simulink model "GolfSwingZVCF"  (R2024b)
settings: Solver=VariableStepAuto  StartTime=0.0  StopTime=StopTime  MaxStep=0.001  RelTol=1e-3
PreLoadFcn:
  | cd(matlabdrive);
  | cd '2DModel';
PostLoadFcn:
  | %run SCRIPT_mdlWksGenerate.m;
  | mdlWks=get_param('GolfSwingZVCF','ModelWorkspace');
  | mdlWks.DataSource = 'MAT-File';
  | mdlWks.FileName = 'ModelInputs.mat';
  | mdlWks.reload;
model workspace: external: MAT-File ModelInputsZVCF.mat (data not in the file)
undefined symbols (not defined in the file): JointTorqueHip, JointTorqueLElbow, JointTorqueLScap, JointTorqueLShoulder, JointTorqueLWrist, JointTorqueRElbow, JointTorqueRScap, JointTorqueRShoulder, JointTorqueRWrist, JointTorqueTorso, X, Y, Z
libraries: nesl_utility x286, sm_lib x176, matrix_library x11, simulink_extras x2
(part 3 of 9)

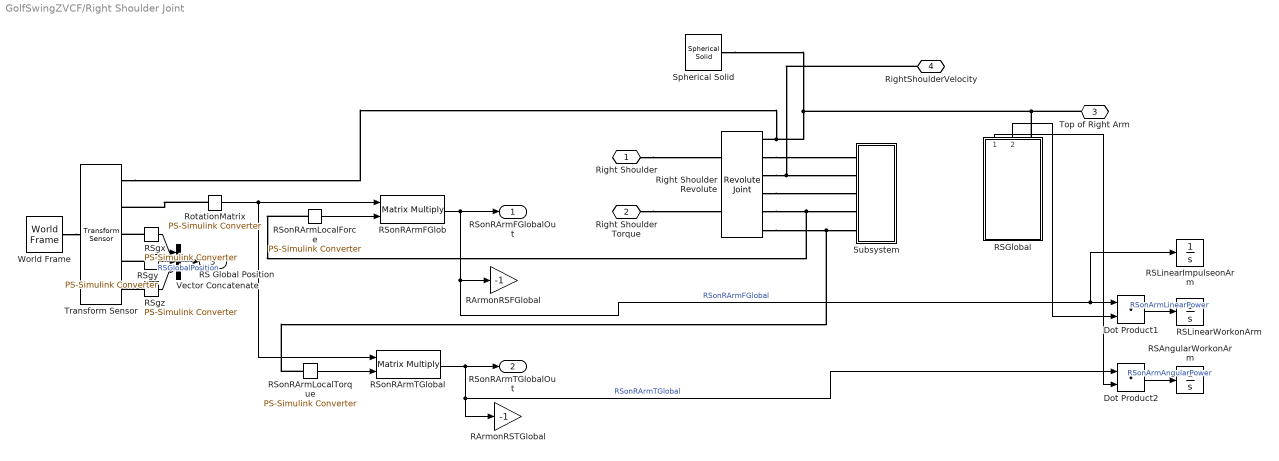
== system GolfSwingZVCF/Right Shoulder Joint ==
  Dot Product1 : DotProduct  OutDataTypeStr=Inherit: Inherit via internal rule
  Dot Product2 : DotProduct  OutDataTypeStr=Inherit: Inherit via internal rule
  RArmonRSFGlobal : Gain  Gain=-1
  RArmonRSTGlobal : Gain  Gain=-1
  RSAngularWorkonArm : Integrator
  RSGlobal : Subsystem
  RSLinearImpulseonArm : Integrator
  RSLinearWorkonArm : Integrator
  RSgx : nesl_utility/PS-Simulink Converter  PhysicalDomain=network_engine_domain  SubClassName=ps_output  LeftPortType=input  RightPortType=output  PseudoPeriodic=off  Frequencies=[]  VectorFormat=1-D array  Unit=inherit  AffineConversion=off
  RSgy : nesl_utility/PS-Simulink Converter  PhysicalDomain=network_engine_domain  SubClassName=ps_output  LeftPortType=input  RightPortType=output  PseudoPeriodic=off  Frequencies=[]  VectorFormat=1-D array  Unit=inherit  AffineConversion=off
  RSgz : nesl_utility/PS-Simulink Converter  PhysicalDomain=network_engine_domain  SubClassName=ps_output  LeftPortType=input  RightPortType=output  PseudoPeriodic=off  Frequencies=[]  VectorFormat=1-D array  Unit=inherit  AffineConversion=off
  RSonRArmFGlob : Product  Multiplication=Matrix(*)
  RSonRArmLocalForce : nesl_utility/PS-Simulink Converter  PhysicalDomain=network_engine_domain  SubClassName=ps_output  LeftPortType=input  RightPortType=output  PseudoPeriodic=off  Frequencies=[]  VectorFormat=1-D array  Unit=inherit  AffineConversion=off
  RSonRArmLocalTorque : nesl_utility/PS-Simulink Converter  PhysicalDomain=network_engine_domain  SubClassName=ps_output  LeftPortType=input  RightPortType=output  PseudoPeriodic=off  Frequencies=[]  VectorFormat=1-D array  Unit=inherit  AffineConversion=off
  RSonRArmTGlobal : Product  Multiplication=Matrix(*)
  Right Shoulder Revolute : sm_lib/Joints/Revolute Joint  JointMode=Normal  CompositeWrenchDir=BaseOnFollower  CompositeWrenchFrame=FollowerFrame  SenseConstraintForce=off  SenseConstraintTorque=off  SenseTotalForce=on  SenseTotalTorque=on  PositionTargetSpecify=on  PositionTargetPriority=Low  PositionTargetValue=RShoulderStartPosition  PositionTargetValueUnits=deg  VelocityTargetSpecify=on  VelocityTargetPriority=High  VelocityTargetValue=RShoulderStartVelocity  VelocityTargetValueUnits=deg/s  EquilibriumPosition=0  EquilibriumPositionUnits=deg  SpringStiffness=0  SpringStiffnessUnits=N*m/deg  DampingCoefficient=0  DampingCoefficientUnits=N*m/(deg/s)  LowerLimitSpecify=off  LowerLimitBound=-150  LowerLimitBoundUnits=deg  LowerLimitStiffness=1e4  LowerLimitStiffnessUnits=N*m/deg  LowerLimitDamping=10  LowerLimitDampingUnits=N*m/(deg/s)  LowerLimitTransitionRegionWidth=0.1  LowerLimitTransitionRegionWidthUnits=deg  UpperLimitSpecify=off  UpperLimitBound=65  UpperLimitBoundUnits=deg  UpperLimitStiffness=1e4  UpperLimitStiffnessUnits=N*m/deg  UpperLimitDamping=10  UpperLimitDampingUnits=N*m/(deg/s)  UpperLimitTransitionRegionWidth=0.1  UpperLimitTransitionRegionWidthUnits=deg  TorqueActuationMode=InputTorque  MotionActuationMode=ComputedMotion  SensePosition=on  SenseVelocity=on  SenseAcceleration=on  SenseTorqueForce=off  SenseLowerLimitTorqueForce=off  SenseUpperLimitTorqueForce=off
      settings: LogSimulationData=on
  RotationMatrix : nesl_utility/PS-Simulink Converter  PhysicalDomain=network_engine_domain  SubClassName=ps_output  LeftPortType=input  RightPortType=output  PseudoPeriodic=off  Frequencies=[]  VectorFormat=1-D array  Unit=inherit  AffineConversion=off
  Spherical Solid : sm_lib/Body Elements/Spherical Solid  SphereRadius=1.75  SphereRadiusUnits=in  ExportEntireGeometry=off  InertiaType=CalculateFromGeometry  BasedOnType=Density  Density=0  DensityUnits=kg/m^3  Mass=1  MassUnits=kg  CenterOfMass=[0 0 0]  CenterOfMassUnits=m  MomentsOfInertia=[1 1 1]  MomentsOfInertiaUnits=kg*m^2  ProductsOfInertia=[0 0 0]  ProductsOfInertiaUnits=kg*m^2  GraphicType=FromGeometry  MarkerShape=Sphere  MarkerSize=10  GraphicVisPropType=SimpleVisualProperties  GraphicDiffuseColor=[0.2 0.2 1.0]  GraphicOpacity=1  GraphicSpecularColor=[0.5 0.5 0.5 1.0]  GraphicAmbientColor=[0.15 0.15 0.15 1.0]  GraphicEmissiveColor=[0.0 0.0 0.0 1.0]  GraphicShininess=75  DoExposeReferenceFrame=on  SerializedFrames=<Frames/>
  Subsystem : Subsystem
  Transform Sensor : sm_lib/Frames and Transforms/Transform Sensor  MeasurementFrame=World  RotationSequence=XYX  SenseAngle=off  SenseAxis=off  SenseQ=off  SenseR=on  SenseRotationSequence=off  SenseOmegaX=off  SenseOmegaY=off  SenseOmegaZ=off  SenseOmega=off  SenseQDot=off  SenseRDot=off  SenseRotationSequenceDot=off  SenseAlphaX=off  SenseAlphaY=off  SenseAlphaZ=off  SenseAlpha=off  SenseQDDot=off  SenseRDDot=off  SenseX=on  SenseY=on  SenseZ=on  SenseXYZ=off  SenseRad=off  SenseAzim=off  SenseDist=off  SenseInc=off  SenseXDot=off  SenseYDot=off  SenseZDot=off  SenseXYZDot=off  SenseRadDot=off  SenseAzimDot=off  SenseDistDot=off  SenseIncDot=off  SenseXDDot=off  SenseYDDot=off  SenseZDDot=off  SenseXYZDDot=off  SenseRadDDot=off  SenseAzimDDot=off  SenseDistDDot=off  SenseIncDDot=off
  Vector Concatenate : Concatenate  NumInputs=3
  World Frame : sm_lib/Frames and Transforms/World Frame
  Right Shoulder : PMIOPort  Side=Left
  Right Shoulder Torque : PMIOPort  Port=2  Side=Left
  Top of Right Arm : PMIOPort  Port=3  Side=Right
  RightShoulderVelocity : PMIOPort  Port=4  Side=Right
  RSonRArmFGlobalOut : Outport
  RSonRArmTGlobalOut : Outport  Port=2
  RS Global Position : Outport  Port=3
  wires:
  RotationMatrix/1 -> RSonRArmFGlob/1, RSonRArmTGlobal/1
  RSonRArmLocalForce/1 -> RSonRArmFGlob/2
  RSonRArmLocalTorque/1 -> RSonRArmTGlobal/2
  RSonRArmTGlobal/1 -> Dot Product2/1, RArmonRSTGlobal/1, RSonRArmTGlobalOut/1  "RSonRArmTGlobal"
  RSgx/1 -> Vector Concatenate/1
  RSgy/1 -> Vector Concatenate/2
  Vector Concatenate/1 -> RS Global Position/1  "RSGlobalPosition"
  RSgz/1 -> Vector Concatenate/3
  Dot Product1/1 -> RSLinearWorkonArm/1  "RSonArmLinearPower"
  Dot Product2/1 -> RSAngularWorkonArm/1  "RSonArmAngularPower"
  RSGlobal/1(RightShoulderGlobalAV) -> Dot Product2/2
  RSGlobal/2(RightShoulderGlobalVelocity) -> Dot Product1/2
  RSonRArmFGlob/1 -> RSLinearImpulseonArm/1, Dot Product1/1, RArmonRSFGlobal/1, RSonRArmFGlobalOut/1  "RSonRArmFGlobal"
  connections:
  Right Shoulder Revolute/RConn6 -- RSonRArmLocalTorque/LConn1 -- Subsystem/LConn5
  Right Shoulder Revolute/RConn4 -- Subsystem/LConn3
  Right Shoulder Revolute/RConn2 -- Subsystem/LConn1
  Right Shoulder Revolute/RConn5 -- RSonRArmLocalForce/LConn1 -- Subsystem/LConn4
  Right Shoulder Revolute/RConn3 -- RightShoulderVelocity/RConn1 -- Subsystem/LConn2
  Right Shoulder Torque/RConn1 -- Right Shoulder Revolute/LConn2
  Right Shoulder/RConn1 -- Right Shoulder Revolute/LConn1
  Spherical Solid/RConn1 -- Top of Right Arm/RConn1 -- RSGlobal/RConn1 -- Transform Sensor/RConn1 -- Right Shoulder Revolute/RConn1
  RSgx/LConn1 -- Transform Sensor/RConn3
  RotationMatrix/LConn1 -- Transform Sensor/RConn2
  RSgz/LConn1 -- Transform Sensor/RConn5
  RSgy/LConn1 -- Transform Sensor/RConn4
  World Frame/RConn1 -- Transform Sensor/LConn1

== system GolfSwingZVCF/Right Upper Arm MOF ==
  RS Global Position : Inport
  RE Global Position : Inport  Port=2
  RSonRArmFGlobalIn : Inport  Port=3
  RSonRArmTGlobalIn : Inport  Port=4
  RForearmonRArmFGlobalIn : Inport  Port=5
  RForearmonRArmTGlobalIn : Inport  Port=6
  R Vector Elbow Force on Right Arm : Sum  Inputs=-+
  R Vector Shoulder Force on Right Arm : Sum  Inputs=-+
  RElbowonRArmMOFGlobal : matrix_library/Cross Product
  RElbowonRArmMOFLocal : Product  Multiplication=Matrix(*)
  RSAngularImpulseonArm : Integrator
  RShoulderonRArmMOFGlobal : matrix_library/Cross Product
  RShoulderonRArmMOFLocal : Product  Multiplication=Matrix(*)
  RUACOM : sm_lib/Body Elements/Inertia Sensor  SensorExtent=BodyGroup  SpanWeldJoints=off  ExcludeGroundedBodies=off  MeasurementFrame=World  SenseMass=off  SenseCenterOfMass=on  SenseInertiaMatrix=off  SenseCenteredInertiaMatrix=off  SensePrincipalInertiaMatrix=off  SenseRotationMatrix=off  GraphicType=None  PrincipalInertiaFrameSize=20  GraphicVisPropType=SimpleVisualProperties  GraphicDiffuseColor=[0.5 0.5 0.5]  GraphicOpacity=1  GraphicSpecularColor=[0.5 0.5 0.5 1.0]  GraphicAmbientColor=[0.15 0.15 0.15 1.0]  GraphicEmissiveColor=[0.0 0.0 0.0 1.0]  GraphicShininess=75
  Right Upper Arm COM : nesl_utility/PS-Simulink Converter  PhysicalDomain=network_engine_domain  SubClassName=ps_output  LeftPortType=input  RightPortType=output  PseudoPeriodic=off  Frequencies=[]  VectorFormat=1-D array  Unit=inherit  AffineConversion=off
  Rotation Transform Right Arm : nesl_utility/PS-Simulink Converter  PhysicalDomain=network_engine_domain  SubClassName=ps_output  LeftPortType=input  RightPortType=output  PseudoPeriodic=off  Frequencies=[]  VectorFormat=1-D array  Unit=inherit  AffineConversion=off
  SumofMomentsRArmLocal : Product  Multiplication=Matrix(*)
  SumofMomentsRSonRArm : Sum
  SumofMomentsRightArmGlobal : Sum  Inputs=++++
  Transform Sensor : sm_lib/Frames and Transforms/Transform Sensor  MeasurementFrame=World  RotationSequence=XYX  SenseAngle=off  SenseAxis=off  SenseQ=off  SenseR=on  SenseRotationSequence=off  SenseOmegaX=off  SenseOmegaY=off  SenseOmegaZ=off  SenseOmega=off  SenseQDot=off  SenseRDot=off  SenseRotationSequenceDot=off  SenseAlphaX=off  SenseAlphaY=off  SenseAlphaZ=off  SenseAlpha=off  SenseQDDot=off  SenseRDDot=off  SenseX=off  SenseY=off  SenseZ=off  SenseXYZ=off  SenseRad=off  SenseAzim=off  SenseDist=off  SenseInc=off  SenseXDot=off  SenseYDot=off  SenseZDot=off  SenseXYZDot=off  SenseRadDot=off  SenseAzimDot=off  SenseDistDot=off  SenseIncDot=off  SenseXDDot=off  SenseYDDot=off  SenseZDDot=off  SenseXYZDDot=off  SenseRadDDot=off  SenseAzimDDot=off  SenseDistDDot=off  SenseIncDDot=off
  World Frame : sm_lib/Frames and Transforms/World Frame
  RightUpper  Arm : PMIOPort  Side=Left
  wires:
  Right Upper Arm COM/1 -> R Vector Elbow Force on Right Arm/1, R Vector Shoulder Force on Right Arm/1  "RUpperArmCOM"
  RS Global Position/1 -> R Vector Shoulder Force on Right Arm/2
  RE Global Position/1 -> R Vector Elbow Force on Right Arm/2
  RSonRArmFGlobalIn/1 -> RShoulderonRArmMOFGlobal/2
  R Vector Elbow Force on Right Arm/1 -> RElbowonRArmMOFGlobal/1
  RForearmonRArmTGlobalIn/1 -> SumofMomentsRightArmGlobal/4
  RForearmonRArmFGlobalIn/1 -> RElbowonRArmMOFGlobal/2
  R Vector Shoulder Force on Right Arm/1 -> RShoulderonRArmMOFGlobal/1
  SumofMomentsRightArmGlobal/1 -> SumofMomentsRArmLocal/2  "SumofMomentsRightArmGlobal"
  RElbowonRArmMOFGlobal/1 -> RElbowonRArmMOFLocal/2, SumofMomentsRightArmGlobal/2  "RElbowonRArmMOFGlobal"
  Rotation Transform Right Arm/1 -> SumofMomentsRArmLocal/1, RElbowonRArmMOFLocal/1, RShoulderonRArmMOFLocal/1
  RShoulderonRArmMOFGlobal/1 -> SumofMomentsRightArmGlobal/1, SumofMomentsRSonRArm/2, RShoulderonRArmMOFLocal/2  "RShoulderonRArmMOFGlobal"
  SumofMomentsRSonRArm/1 -> RSAngularImpulseonArm/1  "SumofMomentsRSonRArm"
  RSonRArmTGlobalIn/1 -> SumofMomentsRSonRArm/1, SumofMomentsRightArmGlobal/3
  connections:
  RUACOM/LConn1 -- Transform Sensor/LConn1 -- RightUpper  Arm/RConn1
  Right Upper Arm COM/LConn1 -- RUACOM/RConn1
  Transform Sensor/RConn1 -- World Frame/RConn1
  Rotation Transform Right Arm/LConn1 -- Transform Sensor/RConn2

== system GolfSwingZVCF/Right Wrist Joint ==
  ClubonRWFGlobal : Gain  Gain=-1
  ClubonRWTGlobal : Gain  Gain=-1
  RWLocalForce : nesl_utility/PS-Simulink Converter  PhysicalDomain=network_engine_domain  SubClassName=ps_output  LeftPortType=input  RightPortType=output  PseudoPeriodic=off  Frequencies=[]  VectorFormat=1-D array  Unit=inherit  AffineConversion=off
  RWLocalTorque : nesl_utility/PS-Simulink Converter  PhysicalDomain=network_engine_domain  SubClassName=ps_output  LeftPortType=input  RightPortType=output  PseudoPeriodic=off  Frequencies=[]  VectorFormat=1-D array  Unit=inherit  AffineConversion=off
  RWgx : nesl_utility/PS-Simulink Converter  PhysicalDomain=network_engine_domain  SubClassName=ps_output  LeftPortType=input  RightPortType=output  PseudoPeriodic=off  Frequencies=[]  VectorFormat=1-D array  Unit=inherit  AffineConversion=off
  RWgy : nesl_utility/PS-Simulink Converter  PhysicalDomain=network_engine_domain  SubClassName=ps_output  LeftPortType=input  RightPortType=output  PseudoPeriodic=off  Frequencies=[]  VectorFormat=1-D array  Unit=inherit  AffineConversion=off
  RWgz : nesl_utility/PS-Simulink Converter  PhysicalDomain=network_engine_domain  SubClassName=ps_output  LeftPortType=input  RightPortType=output  PseudoPeriodic=off  Frequencies=[]  VectorFormat=1-D array  Unit=inherit  AffineConversion=off
  RWonClubFGlobal : Product  Multiplication=Matrix(*)
  RWonClubTGlobal : Product  Multiplication=Matrix(*)
  Right Wrist : sm_lib/Joints/Revolute Joint  JointMode=Normal  CompositeWrenchDir=BaseOnFollower  CompositeWrenchFrame=FollowerFrame  SenseConstraintForce=off  SenseConstraintTorque=off  SenseTotalForce=on  SenseTotalTorque=on  PositionTargetSpecify=off  PositionTargetPriority=Low  PositionTargetValue=70  PositionTargetValueUnits=deg  VelocityTargetSpecify=off  VelocityTargetPriority=Low  VelocityTargetValue=0  VelocityTargetValueUnits=deg/s  EquilibriumPosition=0  EquilibriumPositionUnits=deg  SpringStiffness=0  SpringStiffnessUnits=N*m/deg  DampingCoefficient=0  DampingCoefficientUnits=N*m/(deg/s)  LowerLimitSpecify=off  LowerLimitBound=-90  LowerLimitBoundUnits=deg  LowerLimitStiffness=1e4  LowerLimitStiffnessUnits=N*m/deg  LowerLimitDamping=10  LowerLimitDampingUnits=N*m/(deg/s)  LowerLimitTransitionRegionWidth=0.1  LowerLimitTransitionRegionWidthUnits=deg  UpperLimitSpecify=off  UpperLimitBound=90  UpperLimitBoundUnits=deg  UpperLimitStiffness=1e4  UpperLimitStiffnessUnits=N*m/deg  UpperLimitDamping=10  UpperLimitDampingUnits=N*m/(deg/s)  UpperLimitTransitionRegionWidth=0.1  UpperLimitTransitionRegionWidthUnits=deg  TorqueActuationMode=InputTorque  MotionActuationMode=ComputedMotion  SensePosition=on  SenseVelocity=on  SenseAcceleration=on  SenseTorqueForce=off  SenseLowerLimitTorqueForce=off  SenseUpperLimitTorqueForce=off
      settings: LogSimulationData=on
  RightWristOutputs : Subsystem
  RightWristRelease : Subsystem  Commented=on
  RotationMatrix : nesl_utility/PS-Simulink Converter  PhysicalDomain=network_engine_domain  SubClassName=ps_output  LeftPortType=input  RightPortType=output  PseudoPeriodic=off  Frequencies=[]  VectorFormat=1-D array  Unit=inherit  AffineConversion=off
  Spherical Solid : sm_lib/Body Elements/Spherical Solid  SphereRadius=2  SphereRadiusUnits=in  ExportEntireGeometry=off  InertiaType=CalculateFromGeometry  BasedOnType=Density  Density=0  DensityUnits=kg/m^3  Mass=1  MassUnits=kg  CenterOfMass=[0 0 0]  CenterOfMassUnits=m  MomentsOfInertia=[1 1 1]  MomentsOfInertiaUnits=kg*m^2  ProductsOfInertia=[0 0 0]  ProductsOfInertiaUnits=kg*m^2  GraphicType=FromGeometry  MarkerShape=Sphere  MarkerSize=10  GraphicVisPropType=SimpleVisualProperties  GraphicDiffuseColor=[1.0 0.8 0.4]  GraphicOpacity=1  GraphicSpecularColor=[0.5 0.5 0.5 1.0]  GraphicAmbientColor=[0.15 0.15 0.15 1.0]  GraphicEmissiveColor=[0.0 0.0 0.0 1.0]  GraphicShininess=75  DoExposeReferenceFrame=on  SerializedFrames=<Frames/>
  Transform Sensor1 : sm_lib/Frames and Transforms/Transform Sensor  MeasurementFrame=World  RotationSequence=XYX  SenseAngle=off  SenseAxis=off  SenseQ=off  SenseR=on  SenseRotationSequence=off  SenseOmegaX=off  SenseOmegaY=off  SenseOmegaZ=off  SenseOmega=off  SenseQDot=off  SenseRDot=off  SenseRotationSequenceDot=off  SenseAlphaX=off  SenseAlphaY=off  SenseAlphaZ=off  SenseAlpha=off  SenseQDDot=off  SenseRDDot=off  SenseX=on  SenseY=on  SenseZ=on  SenseXYZ=off  SenseRad=off  SenseAzim=off  SenseDist=off  SenseInc=off  SenseXDot=off  SenseYDot=off  SenseZDot=off  SenseXYZDot=off  SenseRadDot=off  SenseAzimDot=off  SenseDistDot=off  SenseIncDot=off  SenseXDDot=off  SenseYDDot=off  SenseZDDot=off  SenseXYZDDot=off  SenseRadDDot=off  SenseAzimDDot=off  SenseDistDDot=off  SenseIncDDot=off
  Vector Concatenate : Concatenate  NumInputs=3
  World Frame1 : sm_lib/Frames and Transforms/World Frame
  Bottom of Right Forearm : PMIOPort  Side=Left
  RWForce : PMIOPort  Port=2  Side=Right
  RHGrip : PMIOPort  Port=3  Side=Right
  RWTorque : PMIOPort  Port=4  Side=Right
  Right Wrist Torque : PMIOPort  Port=5  Side=Right
  RWVelocity : PMIOPort  Port=6  Side=Right
  RWonClubTGlobalOut : Outport
  RWonClubFGlobalOut : Outport  Port=2
  ClubonRWFGlobalOut : Outport  Port=3
  ClubonRWTGlobalOut : Outport  Port=4
  RWGlobal Position : Outport  Port=5
  wires:
  RWLocalForce/1 -> RWonClubFGlobal/2
  RotationMatrix/1 -> RWonClubTGlobal/1, RWonClubFGlobal/1
  RWLocalTorque/1 -> RWonClubTGlobal/2
  ClubonRWFGlobal/1 -> ClubonRWFGlobalOut/1  "ClubonRWFGlobal"
  RWonClubFGlobal/1 -> ClubonRWFGlobal/1, RWonClubFGlobalOut/1  "RWonClubFGlobal"
  RWonClubTGlobal/1 -> ClubonRWTGlobal/1, RWonClubTGlobalOut/1  "RWonClubTGlobal"
  ClubonRWTGlobal/1 -> ClubonRWTGlobalOut/1  "ClubonRWTGlobal"
  RWgx/1 -> Vector Concatenate/1
  RWgz/1 -> Vector Concatenate/3
  Vector Concatenate/1 -> RWGlobal Position/1  "RWGlobalPosition"
  RWgy/1 -> Vector Concatenate/2
  connections:
  Right Wrist/RConn3 -- RWVelocity/RConn1 -- RightWristOutputs/LConn2
  Bottom of Right Forearm/RConn1 -- Spherical Solid/RConn1 -- Right Wrist/LConn1
  Right Wrist/RConn4 -- RightWristOutputs/LConn3
  Right Wrist/RConn1 -- Transform Sensor1/RConn1 -- RHGrip/RConn1
  Right Wrist/RConn2 -- RightWristOutputs/LConn1
  Right Wrist Torque/RConn1 -- Right Wrist/LConn2
  Right Wrist/RConn5 -- RWLocalForce/LConn1 -- RWForce/RConn1 -- RightWristOutputs/LConn4
  Right Wrist/RConn6 -- RightWristOutputs/LConn5 -- RWLocalTorque/LConn1 -- RWTorque/RConn1
  RotationMatrix/LConn1 -- Transform Sensor1/RConn2
  World Frame1/RConn1 -- Transform Sensor1/LConn1
  Transform Sensor1/RConn4 -- RWgy/LConn1
  Transform Sensor1/RConn5 -- RWgz/LConn1
  Transform Sensor1/RConn3 -- RWgx/LConn1

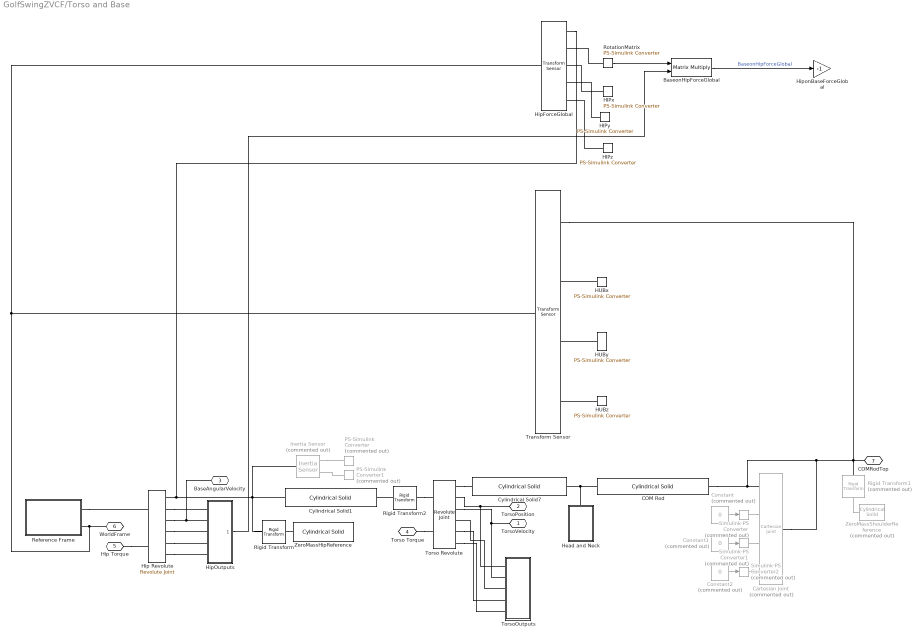
== system GolfSwingZVCF/Torso and Base ==
  BaseonHipForceGlobal : Product  Multiplication=Matrix(*)
  COM Rod : sm_lib/Body Elements/Cylindrical Solid  CylinderRadius=0.1  CylinderRadiusUnits=in  CylinderLength=2  CylinderLengthUnits=in  ExportEntireGeometry=off  InertiaType=CalculateFromGeometry  BasedOnType=Mass  Density=1000  DensityUnits=kg/m^3  Mass=0  MassUnits=kg  CenterOfMass=[0 0 0]  CenterOfMassUnits=m  MomentsOfInertia=[1 1 1]  MomentsOfInertiaUnits=kg*m^2  ProductsOfInertia=[0 0 0]  ProductsOfInertiaUnits=kg*m^2  GraphicType=FromGeometry  MarkerShape=Sphere  MarkerSize=10  GraphicVisPropType=SimpleVisualProperties  GraphicDiffuseColor=[0.5 0.5 0.5]  GraphicOpacity=1.0  GraphicSpecularColor=[0.5 0.5 0.5 1.0]  GraphicAmbientColor=[0.15 0.15 0.15 1.0]  GraphicEmissiveColor=[0.0 0.0 0.0 1.0]  GraphicShininess=75  DoExposeReferenceFrame=off  SerializedFrames=<Frames><Frame><Id>Frame1</Id><Value><Name>COM Rod Bottom</Name><Origin><Source>GeometricFeature</Source><FeatureName>top curve</FeatureName></Origin><PrimaryAxis><DefinedDirection>-X</DefinedDirection><Source>ReferenceFrame</Source><SourceDirection>-Y</SourceDirection><FeatureName></FeatureName></PrimaryAxis><SecondaryAxis><DefinedDirection>+Y</DefinedDirection><Source>ReferenceFrame</Source><SourceDirection>+Z</SourceDirection><FeatureName></FeatureName></SecondaryAxis></Value></Frame><Frame><Id>Frame2</Id><Value><Name>COM Rod Top</Name><Origin><Source>GeometricFeature</Source><FeatureName>bottom curve</FeatureName></Origin><PrimaryAxis><DefinedDirection>+X</DefinedDirection><Source>ReferenceFrame</Source><SourceDirection>+Y</SourceDirection><FeatureName></FeatureName></PrimaryAxis><SecondaryAxis><DefinedDirection>+Y</DefinedDirection><Source>ReferenceFrame</Source><SourceDirection>-Z</SourceDirection><FeatureName></FeatureName></SecondaryAxis></Value></Frame></Frames>
  Cartesian Joint : sm_lib/Joints/Cartesian Joint  Commented=on  JointMode=Normal  CompositeWrenchDir=FollowerOnBase  CompositeWrenchFrame=BaseFrame  SenseConstraintForce=off  SenseConstraintTorque=off  SenseTotalForce=off  SenseTotalTorque=off  PxPositionTargetSpecify=off  PxPositionTargetPriority=High  PxPositionTargetValue=0  PxPositionTargetValueUnits=m  PxVelocityTargetSpecify=off  PxVelocityTargetPriority=High  PxVelocityTargetValue=0  PxVelocityTargetValueUnits=m/s  PxEquilibriumPosition=0  PxEquilibriumPositionUnits=m  PxSpringStiffness=100  PxSpringStiffnessUnits=N/m  PxDampingCoefficient=10  PxDampingCoefficientUnits=N/(m/s)  PxLowerLimitSpecify=off  PxLowerLimitBound=-1  PxLowerLimitBoundUnits=m  PxLowerLimitStiffness=1e6  PxLowerLimitStiffnessUnits=N/m  PxLowerLimitDamping=1e3  PxLowerLimitDampingUnits=N/(m/s)  PxLowerLimitTransitionRegionWidth=1e-4  PxLowerLimitTransitionRegionWidthUnits=m  PxUpperLimitSpecify=off  PxUpperLimitBound=1  PxUpperLimitBoundUnits=m  PxUpperLimitStiffness=1e6  PxUpperLimitStiffnessUnits=N/m  PxUpperLimitDamping=1e3  PxUpperLimitDampingUnits=N/(m/s)  PxUpperLimitTransitionRegionWidth=1e-4  PxUpperLimitTransitionRegionWidthUnits=m  PxTorqueActuationMode=InputTorque  PxMotionActuationMode=ComputedMotion  PxSensePosition=off  PxSenseVelocity=off  PxSenseAcceleration=off  PxSenseTorqueForce=off  PxSenseLowerLimitTorqueForce=off  PxSenseUpperLimitTorqueForce=off  PyPositionTargetSpecify=off  PyPositionTargetPriority=High  PyPositionTargetValue=0  PyPositionTargetValueUnits=m  PyVelocityTargetSpecify=off  PyVelocityTargetPriority=High  PyVelocityTargetValue=0  PyVelocityTargetValueUnits=m/s  PyEquilibriumPosition=0  PyEquilibriumPositionUnits=m  PySpringStiffness=100  PySpringStiffnessUnits=N/m  PyDampingCoefficient=10  PyDampingCoefficientUnits=N/(m/s)  PyLowerLimitSpecify=off  PyLowerLimitBound=-1  PyLowerLimitBoundUnits=m  PyLowerLimitStiffness=1e6  PyLowerLimitStiffnessUnits=N/m  PyLowerLimitDamping=1e3  PyLowerLimitDampingUnits=N/(m/s)  PyLowerLimitTransitionRegionWidth=1e-4  PyLowerLimitTransitionRegionWidthUnits=m  PyUpperLimitSpecify=off  PyUpperLimitBound=1  PyUpperLimitBoundUnits=m  PyUpperLimitStiffness=1e6  PyUpperLimitStiffnessUnits=N/m  PyUpperLimitDamping=1e3  PyUpperLimitDampingUnits=N/(m/s)  PyUpperLimitTransitionRegionWidth=1e-4  PyUpperLimitTransitionRegionWidthUnits=m  PyTorqueActuationMode=InputTorque  PyMotionActuationMode=ComputedMotion  PySensePosition=off  PySenseVelocity=off  PySenseAcceleration=off  PySenseTorqueForce=off  PySenseLowerLimitTorqueForce=off  PySenseUpperLimitTorqueForce=off  PzPositionTargetSpecify=off  PzPositionTargetPriority=High  PzPositionTargetValue=0  PzPositionTargetValueUnits=m  PzVelocityTargetSpecify=off  PzVelocityTargetPriority=High  PzVelocityTargetValue=0  PzVelocityTargetValueUnits=m/s  PzEquilibriumPosition=0  PzEquilibriumPositionUnits=m  PzSpringStiffness=100  PzSpringStiffnessUnits=N/m  PzDampingCoefficient=10  PzDampingCoefficientUnits=N/(m/s)  PzLowerLimitSpecify=off  PzLowerLimitBound=-1  PzLowerLimitBoundUnits=m  PzLowerLimitStiffness=1e6  PzLowerLimitStiffnessUnits=N/m  PzLowerLimitDamping=1e3  PzLowerLimitDampingUnits=N/(m/s)  PzLowerLimitTransitionRegionWidth=1e-4  PzLowerLimitTransitionRegionWidthUnits=m  PzUpperLimitSpecify=off  PzUpperLimitBound=1  PzUpperLimitBoundUnits=m  PzUpperLimitStiffness=1e6  PzUpperLimitStiffnessUnits=N/m  PzUpperLimitDamping=1e3  PzUpperLimitDampingUnits=N/(m/s)  PzUpperLimitTransitionRegionWidth=1e-4  PzUpperLimitTransitionRegionWidthUnits=m  PzTorqueActuationMode=InputTorque  PzMotionActuationMode=ComputedMotion  PzSensePosition=off  PzSenseVelocity=off  PzSenseAcceleration=off  PzSenseTorqueForce=off  PzSenseLowerLimitTorqueForce=off  PzSenseUpperLimitTorqueForce=off
  Constant : Constant  Commented=on  Value=0
  Constant1 : Constant  Commented=on  Value=0
  Constant2 : Constant  Commented=on  Value=0
  Cylindrical Solid1 : sm_lib/Body Elements/Cylindrical Solid  CylinderRadius=6  CylinderRadiusUnits=in  CylinderLength=15  CylinderLengthUnits=in  ExportEntireGeometry=off  InertiaType=CalculateFromGeometry  BasedOnType=Mass  Density=1000  DensityUnits=kg/m^3  Mass=20  MassUnits=kg  CenterOfMass=[0 0 0]  CenterOfMassUnits=m  MomentsOfInertia=[1 1 1]  MomentsOfInertiaUnits=kg*m^2  ProductsOfInertia=[0 0 0]  ProductsOfInertiaUnits=kg*m^2  GraphicType=FromGeometry  MarkerShape=Sphere  MarkerSize=10  GraphicVisPropType=SimpleVisualProperties  GraphicDiffuseColor=[0.2 0.2 0.0]  GraphicOpacity=1.0  GraphicSpecularColor=[0.5 0.5 0.5 1.0]  GraphicAmbientColor=[0.15 0.15 0.15 1.0]  GraphicEmissiveColor=[0.0 0.0 0.0 1.0]  GraphicShininess=75  DoExposeReferenceFrame=off  SerializedFrames=<Frames><Frame><Id>Frame1</Id><Value><Name>Bottom of Hips</Name><Origin><Source>GeometricFeature</Source><FeatureName>top surface</FeatureName></Origin><PrimaryAxis><DefinedDirection>-Z</DefinedDirection><Source>ReferenceFrame</Source><SourceDirection>+Z</SourceDirection><FeatureName></FeatureName></PrimaryAxis><SecondaryAxis><DefinedDirection>+X</DefinedDirection><Source>ReferenceFrame</Source><SourceDirection>+X</SourceDirection><FeatureName></FeatureName></SecondaryAxis></Value></Frame><Frame><Id>Frame2</Id><Value><Name>Top of Hips</Name><Origin><Source>GeometricFeature</Source><FeatureName>bottom surface</FeatureName></Origin><PrimaryAxis><DefinedDirection>+Z</DefinedDirection><Source>ReferenceFrame</Source><SourceDirection>+Z</SourceDirection><FeatureName></FeatureName></PrimaryAxis><SecondaryAxis><DefinedDirection>+X</DefinedDirection><Source>ReferenceFrame</Source><SourceDirection>+X</SourceDirection><FeatureName></FeatureName></SecondaryAxis></Value></Frame></Frames>
  Cylindrical Solid7 : sm_lib/Body Elements/Cylindrical Solid  CylinderRadius=6  CylinderRadiusUnits=in  CylinderLength=15  CylinderLengthUnits=in  ExportEntireGeometry=off  InertiaType=CalculateFromGeometry  BasedOnType=Mass  Density=1000  DensityUnits=kg/m^3  Mass=20  MassUnits=kg  CenterOfMass=[0 0 0]  CenterOfMassUnits=m  MomentsOfInertia=[1 1 1]  MomentsOfInertiaUnits=kg*m^2  ProductsOfInertia=[0 0 0]  ProductsOfInertiaUnits=kg*m^2  GraphicType=FromGeometry  MarkerShape=Sphere  MarkerSize=10  GraphicVisPropType=SimpleVisualProperties  GraphicDiffuseColor=[0.2 0.2 1.0]  GraphicOpacity=1.0  GraphicSpecularColor=[0.5 0.5 0.5 1.0]  GraphicAmbientColor=[0.15 0.15 0.15 1.0]  GraphicEmissiveColor=[0.0 0.0 0.0 1.0]  GraphicShininess=75  DoExposeReferenceFrame=off  SerializedFrames=<Frames><Frame><Id>Frame1</Id><Value><Name>Bottom of Torso</Name><Origin><Source>GeometricFeature</Source><FeatureName>top surface</FeatureName></Origin><PrimaryAxis><DefinedDirection>-Z</DefinedDirection><Source>ReferenceFrame</Source><SourceDirection>+Z</SourceDirection><FeatureName></FeatureName></PrimaryAxis><SecondaryAxis><DefinedDirection>+X</DefinedDirection><Source>ReferenceFrame</Source><SourceDirection>+X</SourceDirection><FeatureName></FeatureName></SecondaryAxis></Value></Frame><Frame><Id>Frame2</Id><Value><Name>Top of Torso</Name><Origin><Source>GeometricFeature</Source><FeatureName>bottom surface</FeatureName></Origin><PrimaryAxis><DefinedDirection>+Z</DefinedDirection><Source>ReferenceFrame</Source><SourceDirection>+Z</SourceDirection><FeatureName></FeatureName></PrimaryAxis><SecondaryAxis><DefinedDirection>+X</DefinedDirection><Source>ReferenceFrame</Source><SourceDirection>+X</SourceDirection><FeatureName></FeatureName></SecondaryAxis></Value></Frame></Frames>
  HIPx : nesl_utility/PS-Simulink Converter  PhysicalDomain=network_engine_domain  SubClassName=ps_output  LeftPortType=input  RightPortType=output  PseudoPeriodic=off  Frequencies=[]  VectorFormat=1-D array  Unit=inherit  AffineConversion=off
  HIPy : nesl_utility/PS-Simulink Converter  PhysicalDomain=network_engine_domain  SubClassName=ps_output  LeftPortType=input  RightPortType=output  PseudoPeriodic=off  Frequencies=[]  VectorFormat=1-D array  Unit=inherit  AffineConversion=off
  HIPz : nesl_utility/PS-Simulink Converter  PhysicalDomain=network_engine_domain  SubClassName=ps_output  LeftPortType=input  RightPortType=output  PseudoPeriodic=off  Frequencies=[]  VectorFormat=1-D array  Unit=inherit  AffineConversion=off
  HUBx : nesl_utility/PS-Simulink Converter  PhysicalDomain=network_engine_domain  SubClassName=ps_output  LeftPortType=input  RightPortType=output  PseudoPeriodic=off  Frequencies=[]  VectorFormat=1-D array  Unit=inherit  AffineConversion=off
  HUBy : nesl_utility/PS-Simulink Converter  PhysicalDomain=network_engine_domain  SubClassName=ps_output  LeftPortType=input  RightPortType=output  PseudoPeriodic=off  Frequencies=[]  VectorFormat=1-D array  Unit=inherit  AffineConversion=off
  HUBz : nesl_utility/PS-Simulink Converter  PhysicalDomain=network_engine_domain  SubClassName=ps_output  LeftPortType=input  RightPortType=output  PseudoPeriodic=off  Frequencies=[]  VectorFormat=1-D array  Unit=inherit  AffineConversion=off
  Head and Neck : Subsystem
      settings: PortSchema="{\"entries\":[{\"content\":{\"sides\":[{\"content\":{\"connectorIds\":[]},\"type\":\"ConnectorPlacement.EquallySpacedRectSide\",\"uuid\":\"f3d48692-b84b-459b-b36d-09e850943f16\"},{\"content\":{\"connectorIds\":[],\"side\":\"RIGHT\"},\"type\":\"ConnectorPlacement.EquallySpacedRectSide\",\"uuid\":\"ca17451e-58c8-4f5d-a171-c34bc8bcba56\"},{\"content\":{\"connectorIds\":[\"LConn1\"],\"side\":\"TOP\"},\"type\":\"ConnectorPlacement.EquallySpacedRectSide\",\"uuid\":\"7a785aaf-dbfc-4452-a340-00487f390d44\"}]},\"type\":\"ConnectorPlacement.EquallySpacedConnector\",\"uuid\":\"64da2f62-4262-44eb-a378-0f3b9a710057\"}],\"packageUris\":[\"http://schema.mathworks.com/mf0/Connector/R2020b\"],\"version\":\"1.0\"}"
  Hip Revolute : sm_lib/Joints/Revolute Joint  JointMode=Normal  CompositeWrenchDir=BaseOnFollower  CompositeWrenchFrame=FollowerFrame  SenseConstraintForce=off  SenseConstraintTorque=off  SenseTotalForce=on  SenseTotalTorque=on  PositionTargetSpecify=on  PositionTargetPriority=High  PositionTargetValue=HipStartPosition  PositionTargetValueUnits=deg  VelocityTargetSpecify=on  VelocityTargetPriority=High  VelocityTargetValue=HipStartVelocity  VelocityTargetValueUnits=deg/s  EquilibriumPosition=0  EquilibriumPositionUnits=deg  SpringStiffness=0  SpringStiffnessUnits=N*m/deg  DampingCoefficient=0  DampingCoefficientUnits=N*m/(deg/s)  LowerLimitSpecify=off  LowerLimitBound=-90  LowerLimitBoundUnits=deg  LowerLimitStiffness=1e4  LowerLimitStiffnessUnits=N*m/deg  LowerLimitDamping=10  LowerLimitDampingUnits=N*m/(deg/s)  LowerLimitTransitionRegionWidth=0.1  LowerLimitTransitionRegionWidthUnits=deg  UpperLimitSpecify=off  UpperLimitBound=90  UpperLimitBoundUnits=deg  UpperLimitStiffness=1e4  UpperLimitStiffnessUnits=N*m/deg  UpperLimitDamping=10  UpperLimitDampingUnits=N*m/(deg/s)  UpperLimitTransitionRegionWidth=0.1  UpperLimitTransitionRegionWidthUnits=deg  TorqueActuationMode=InputTorque  MotionActuationMode=ComputedMotion  SensePosition=on  SenseVelocity=on  SenseAcceleration=on  SenseTorqueForce=off  SenseLowerLimitTorqueForce=off  SenseUpperLimitTorqueForce=off
  HipForceGlobal : sm_lib/Frames and Transforms/Transform Sensor  MeasurementFrame=World  RotationSequence=XYX  SenseAngle=off  SenseAxis=off  SenseQ=off  SenseR=on  SenseRotationSequence=off  SenseOmegaX=off  SenseOmegaY=off  SenseOmegaZ=off  SenseOmega=off  SenseQDot=off  SenseRDot=off  SenseRotationSequenceDot=off  SenseAlphaX=off  SenseAlphaY=off  SenseAlphaZ=off  SenseAlpha=off  SenseQDDot=off  SenseRDDot=off  SenseX=on  SenseY=on  SenseZ=on  SenseXYZ=off  SenseRad=off  SenseAzim=off  SenseDist=off  SenseInc=off  SenseXDot=off  SenseYDot=off  SenseZDot=off  SenseXYZDot=off  SenseRadDot=off  SenseAzimDot=off  SenseDistDot=off  SenseIncDot=off  SenseXDDot=off  SenseYDDot=off  SenseZDDot=off  SenseXYZDDot=off  SenseRadDDot=off  SenseAzimDDot=off  SenseDistDDot=off  SenseIncDDot=off
  HipOutputs : Subsystem
  HiponBaseForceGlobal : Gain  Gain=-1
  Inertia Sensor : sm_lib/Body Elements/Inertia Sensor  Commented=on  SensorExtent=Mechanism  SpanWeldJoints=off  ExcludeGroundedBodies=off  MeasurementFrame=World  SenseMass=on  SenseCenterOfMass=on  SenseInertiaMatrix=off  SenseCenteredInertiaMatrix=off  SensePrincipalInertiaMatrix=off  SenseRotationMatrix=off  GraphicType=None  PrincipalInertiaFrameSize=20  GraphicVisPropType=SimpleVisualProperties  GraphicDiffuseColor=[0.5 0.5 0.5]  GraphicOpacity=1  GraphicSpecularColor=[0.5 0.5 0.5 1.0]  GraphicAmbientColor=[0.15 0.15 0.15 1.0]  GraphicEmissiveColor=[0.0 0.0 0.0 1.0]  GraphicShininess=75
  PS-Simulink Converter : nesl_utility/PS-Simulink Converter  Commented=on  PhysicalDomain=network_engine_domain  SubClassName=ps_output  LeftPortType=input  RightPortType=output  PseudoPeriodic=off  Frequencies=[]  VectorFormat=1-D array  Unit=inherit  AffineConversion=off
  PS-Simulink Converter1 : nesl_utility/PS-Simulink Converter  Commented=on  PhysicalDomain=network_engine_domain  SubClassName=ps_output  LeftPortType=input  RightPortType=output  PseudoPeriodic=off  Frequencies=[]  VectorFormat=1-D array  Unit=inherit  AffineConversion=off
  Reference Frame : Subsystem
  Rigid Transform : sm_lib/Frames and Transforms/Rigid Transform  RotationMethod=RotationSequence  FollAlignAxisA=+X  BaseAlignAxisA=+Y  FollAlignAxisB=+Y  BaseAlignAxisB=+Z  RotationStandardAxis=+Z  RotationAngle=0.0  RotationAngleUnits=deg  RotationArbitraryAxis=[0 0 1]  RotationSequenceAxes=BaseAxes  RotationSequence=XYX  RotationSequenceAngles=[0 90 0]  RotationSequenceAnglesUnits=deg  RotationMatrix=[1 0 0; 0 1 0; 0 0 1]  Quaternion=[1 0 0 0]  TranslationMethod=None  TranslationCartesianOffset=[0 0 0]  TranslationCartesianOffsetUnits=m  TranslationStandardAxis=+Z  TranslationStandardOffset=0  TranslationStandardOffsetUnits=m  TranslationROffset=0  TranslationROffsetUnits=m  TranslationThetaOffset=0  TranslationThetaOffsetUnits=deg  TranslationZOffset=0  TranslationZOffsetUnits=m
  Rigid Transform1 : sm_lib/Frames and Transforms/Rigid Transform  Commented=on  RotationMethod=RotationSequence  FollAlignAxisA=+X  BaseAlignAxisA=+Y  FollAlignAxisB=+Y  BaseAlignAxisB=+Z  RotationStandardAxis=+Z  RotationAngle=0.0  RotationAngleUnits=deg  RotationArbitraryAxis=[0 0 1]  RotationSequenceAxes=BaseAxes  RotationSequence=XYX  RotationSequenceAngles=[0 90 0]  RotationSequenceAnglesUnits=deg  RotationMatrix=[1 0 0; 0 1 0; 0 0 1]  Quaternion=[1 0 0 0]  TranslationMethod=None  TranslationCartesianOffset=[0 0 0]  TranslationCartesianOffsetUnits=m  TranslationStandardAxis=+Z  TranslationStandardOffset=0  TranslationStandardOffsetUnits=m  TranslationROffset=0  TranslationROffsetUnits=m  TranslationThetaOffset=0  TranslationThetaOffsetUnits=deg  TranslationZOffset=0  TranslationZOffsetUnits=m
  Rigid Transform2 : sm_lib/Frames and Transforms/Rigid Transform  RotationMethod=RotationSequence  FollAlignAxisA=+X  BaseAlignAxisA=+Y  FollAlignAxisB=+Y  BaseAlignAxisB=+Z  RotationStandardAxis=+Z  RotationAngle=0.0  RotationAngleUnits=deg  RotationArbitraryAxis=[0 0 1]  RotationSequenceAxes=BaseAxes  RotationSequence=XYZ  RotationSequenceAngles=[180 0 0]  RotationSequenceAnglesUnits=deg  RotationMatrix=[1 0 0; 0 1 0; 0 0 1]  Quaternion=[1 0 0 0]  TranslationMethod=None  TranslationCartesianOffset=[0 0 0]  TranslationCartesianOffsetUnits=m  TranslationStandardAxis=+Z  TranslationStandardOffset=0  TranslationStandardOffsetUnits=m  TranslationROffset=0  TranslationROffsetUnits=m  TranslationThetaOffset=0  TranslationThetaOffsetUnits=deg  TranslationZOffset=0  TranslationZOffsetUnits=m
  RotationMatrix : nesl_utility/PS-Simulink Converter  PhysicalDomain=network_engine_domain  SubClassName=ps_output  LeftPortType=input  RightPortType=output  PseudoPeriodic=off  Frequencies=[]  VectorFormat=1-D array  Unit=inherit  AffineConversion=off
  Simulink-PS Converter : nesl_utility/Simulink-PS Converter  Commented=on  PhysicalDomain=network_engine_domain  SubClassName=ps_input  LeftPortType=input  RightPortType=output  PseudoPeriodic=off  Frequencies=[]  NoiseDistribution=none  NoiseParameters=[]  Unit=1  AffineConversion=off  FilteringAndDerivatives=provide  SimscapeFilterOrder=1  InputFilterTimeConstant=0.001  UdotUserProvided=0
  Simulink-PS Converter1 : nesl_utility/Simulink-PS Converter  Commented=on  PhysicalDomain=network_engine_domain  SubClassName=ps_input  LeftPortType=input  RightPortType=output  PseudoPeriodic=off  Frequencies=[]  NoiseDistribution=none  NoiseParameters=[]  Unit=1  AffineConversion=off  FilteringAndDerivatives=provide  SimscapeFilterOrder=1  InputFilterTimeConstant=0.001  UdotUserProvided=0
  Simulink-PS Converter2 : nesl_utility/Simulink-PS Converter  Commented=on  PhysicalDomain=network_engine_domain  SubClassName=ps_input  LeftPortType=input  RightPortType=output  PseudoPeriodic=off  Frequencies=[]  NoiseDistribution=none  NoiseParameters=[]  Unit=1  AffineConversion=off  FilteringAndDerivatives=provide  SimscapeFilterOrder=1  InputFilterTimeConstant=0.001  UdotUserProvided=0
  Torso Revolute : sm_lib/Joints/Revolute Joint  JointMode=Normal  CompositeWrenchDir=BaseOnFollower  CompositeWrenchFrame=FollowerFrame  SenseConstraintForce=off  SenseConstraintTorque=off  SenseTotalForce=on  SenseTotalTorque=on  PositionTargetSpecify=on  PositionTargetPriority=High  PositionTargetValue=TorsoStartPosition  PositionTargetValueUnits=deg  VelocityTargetSpecify=on  VelocityTargetPriority=High  VelocityTargetValue=TorsoStartVelocity  VelocityTargetValueUnits=deg/s  EquilibriumPosition=-65  EquilibriumPositionUnits=deg  SpringStiffness=0  SpringStiffnessUnits=N*m/deg  DampingCoefficient=0  DampingCoefficientUnits=N*m/(deg/s)  LowerLimitSpecify=off  LowerLimitBound=-65  LowerLimitBoundUnits=deg  LowerLimitStiffness=4  LowerLimitStiffnessUnits=N*m/deg  LowerLimitDamping=0.1  LowerLimitDampingUnits=N*m/(deg/s)  LowerLimitTransitionRegionWidth=10  LowerLimitTransitionRegionWidthUnits=deg  UpperLimitSpecify=off  UpperLimitBound=65  UpperLimitBoundUnits=deg  UpperLimitStiffness=4  UpperLimitStiffnessUnits=N*m/deg  UpperLimitDamping=0.1  UpperLimitDampingUnits=N*m/(deg/s)  UpperLimitTransitionRegionWidth=10  UpperLimitTransitionRegionWidthUnits=deg  TorqueActuationMode=InputTorque  MotionActuationMode=ComputedMotion  SensePosition=on  SenseVelocity=on  SenseAcceleration=on  SenseTorqueForce=off  SenseLowerLimitTorqueForce=off  SenseUpperLimitTorqueForce=off
  TorsoOutputs : Subsystem
  Transform Sensor : sm_lib/Frames and Transforms/Transform Sensor  MeasurementFrame=World  RotationSequence=XYX  SenseAngle=off  SenseAxis=off  SenseQ=off  SenseR=off  SenseRotationSequence=off  SenseOmegaX=off  SenseOmegaY=off  SenseOmegaZ=off  SenseOmega=off  SenseQDot=off  SenseRDot=off  SenseRotationSequenceDot=off  SenseAlphaX=off  SenseAlphaY=off  SenseAlphaZ=off  SenseAlpha=off  SenseQDDot=off  SenseRDDot=off  SenseX=on  SenseY=on  SenseZ=on  SenseXYZ=off  SenseRad=off  SenseAzim=off  SenseDist=off  SenseInc=off  SenseXDot=off  SenseYDot=off  SenseZDot=off  SenseXYZDot=off  SenseRadDot=off  SenseAzimDot=off  SenseDistDot=off  SenseIncDot=off  SenseXDDot=off  SenseYDDot=off  SenseZDDot=off  SenseXYZDDot=off  SenseRadDDot=off  SenseAzimDDot=off  SenseDistDDot=off  SenseIncDDot=off
  ZeroMassHipReference : sm_lib/Body Elements/Cylindrical Solid  CylinderRadius=4  CylinderRadiusUnits=in  CylinderLength=12  CylinderLengthUnits=in  ExportEntireGeometry=off  InertiaType=CalculateFromGeometry  BasedOnType=Mass  Density=1000  DensityUnits=kg/m^3  Mass=0  MassUnits=kg  CenterOfMass=[0 0 0]  CenterOfMassUnits=m  MomentsOfInertia=[1 1 1]  MomentsOfInertiaUnits=kg*m^2  ProductsOfInertia=[0 0 0]  ProductsOfInertiaUnits=kg*m^2  GraphicType=FromGeometry  MarkerShape=Sphere  MarkerSize=10  GraphicVisPropType=SimpleVisualProperties  GraphicDiffuseColor=[0.2 0.2 0.0]  GraphicOpacity=1.0  GraphicSpecularColor=[0.5 0.5 0.5 1.0]  GraphicAmbientColor=[0.15 0.15 0.15 1.0]  GraphicEmissiveColor=[0.0 0.0 0.0 1.0]  GraphicShininess=75  DoExposeReferenceFrame=on  SerializedFrames=<Frames/>
  ZeroMassShoulderReference : sm_lib/Body Elements/Cylindrical Solid  Commented=on  CylinderRadius=4  CylinderRadiusUnits=in  CylinderLength=12  CylinderLengthUnits=in  ExportEntireGeometry=off  InertiaType=CalculateFromGeometry  BasedOnType=Mass  Density=1000  DensityUnits=kg/m^3  Mass=0  MassUnits=kg  CenterOfMass=[0 0 0]  CenterOfMassUnits=m  MomentsOfInertia=[1 1 1]  MomentsOfInertiaUnits=kg*m^2  ProductsOfInertia=[0 0 0]  ProductsOfInertiaUnits=kg*m^2  GraphicType=FromGeometry  MarkerShape=Sphere  MarkerSize=10  GraphicVisPropType=SimpleVisualProperties  GraphicDiffuseColor=[0.6 1.0 1.0]  GraphicOpacity=1.0  GraphicSpecularColor=[0.5 0.5 0.5 1.0]  GraphicAmbientColor=[0.15 0.15 0.15 1.0]  GraphicEmissiveColor=[0.0 0.0 0.0 1.0]  GraphicShininess=75  DoExposeReferenceFrame=on  SerializedFrames=<Frames/>
  TorsoVelocity : PMIOPort  Side=Left
  TorsoPosition : PMIOPort  Port=2  Side=Left
  BaseAngularVelocity : PMIOPort  Port=3  Side=Left
  Torso Torque : PMIOPort  Port=4  Side=Right
  Hip Torque : PMIOPort  Port=5  Side=Right
  WorldFrame : PMIOPort  Port=6  Side=Right
  COMRodTop : PMIOPort  Port=7  Side=Right
  wires:
  Constant1/1 -> Simulink-PS Converter1/1
  Constant2/1 -> Simulink-PS Converter2/1
  Constant/1 -> Simulink-PS Converter/1
  HipOutputs/1(HipForceOut) -> BaseonHipForceGlobal/2
  RotationMatrix/1 -> BaseonHipForceGlobal/1
  BaseonHipForceGlobal/1 -> HiponBaseForceGlobal/1  "BaseonHipForceGlobal"
  connections:
  Torso Revolute/RConn3 -- TorsoOutputs/LConn2 -- TorsoVelocity/RConn1
  Rigid Transform1/LConn1 -- ZeroMassShoulderReference/RConn1
  COM Rod/RConn1 -- Cartesian Joint/RConn1 -- Transform Sensor/RConn1 -- Rigid Transform1/RConn1 -- COMRodTop/RConn1 -- Cartesian Joint/LConn1
  TorsoOutputs/LConn3 -- Torso Revolute/RConn4
  Torso Revolute/RConn2 -- TorsoOutputs/LConn1 -- TorsoPosition/RConn1
  Reference Frame/RConn2 -- HipForceGlobal/LConn1 -- Transform Sensor/LConn1 -- WorldFrame/RConn1
  Rigid Transform/LConn1 -- ZeroMassHipReference/RConn1
  Hip Revolute/RConn1 -- HipForceGlobal/RConn1 -- Inertia Sensor/LConn1 -- Rigid Transform/RConn1 -- Cylindrical Solid1/LConn1
  Torso Revolute/RConn1 -- Cylindrical Solid7/LConn1
  Torso Torque/RConn1 -- Torso Revolute/LConn2
  Hip Torque/RConn1 -- Hip Revolute/LConn2
  Reference Frame/RConn1 -- Hip Revolute/LConn1
  Hip Revolute/RConn6 -- HipOutputs/LConn5
  Hip Revolute/RConn2 -- HipOutputs/LConn1
  Hip Revolute/RConn3 -- BaseAngularVelocity/RConn1 -- HipOutputs/LConn2
  Hip Revolute/RConn4 -- HipOutputs/LConn3
  Hip Revolute/RConn5 -- HipOutputs/LConn4
  COM Rod/LConn1 -- Head and Neck/LConn1 -- Cylindrical Solid7/RConn1
  Rigid Transform2/LConn1 -- Cylindrical Solid1/RConn1
  Rigid Transform2/RConn1 -- Torso Revolute/LConn1
  Torso Revolute/RConn6 -- TorsoOutputs/LConn5
  Torso Revolute/RConn5 -- TorsoOutputs/LConn4
  Simulink-PS Converter2/RConn1 -- Cartesian Joint/LConn4
  Simulink-PS Converter/RConn1 -- Cartesian Joint/LConn2
  Simulink-PS Converter1/RConn1 -- Cartesian Joint/LConn3
  HUBx/LConn1 -- Transform Sensor/RConn2
  HUBz/LConn1 -- Transform Sensor/RConn4
  HUBy/LConn1 -- Transform Sensor/RConn3
  Inertia Sensor/RConn1 -- PS-Simulink Converter/LConn1
  PS-Simulink Converter1/LConn1 -- Inertia Sensor/RConn2
  HIPz/LConn1 -- HipForceGlobal/RConn5
  RotationMatrix/LConn1 -- HipForceGlobal/RConn2
  HIPx/LConn1 -- HipForceGlobal/RConn3
  HIPy/LConn1 -- HipForceGlobal/RConn4

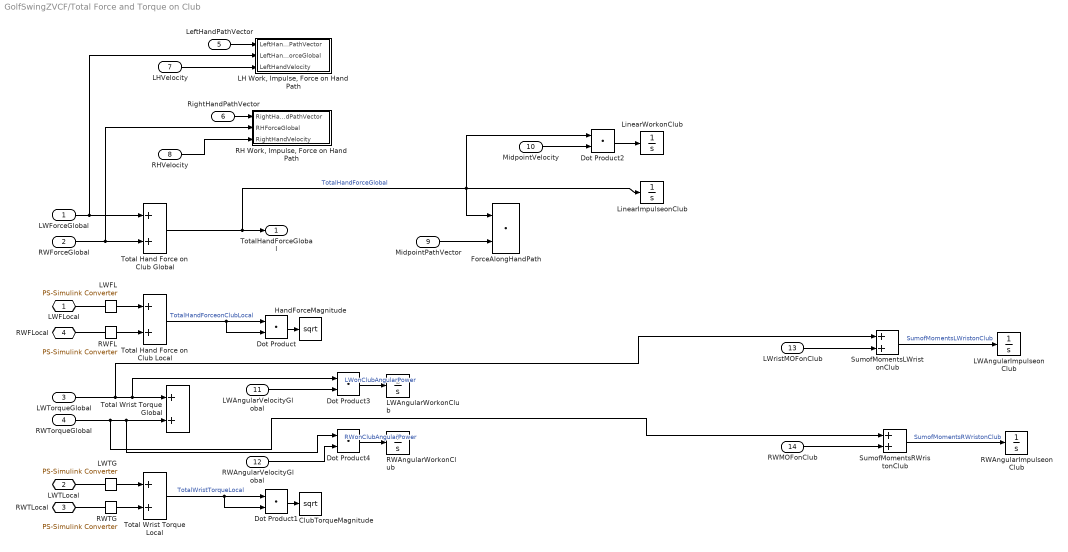
== system GolfSwingZVCF/Total Force and Torque on Club ==
  LWForceGlobal : Inport
  RWForceGlobal : Inport  Port=2
  LWTorqueGlobal : Inport  Port=3
  RWTorqueGlobal : Inport  Port=4
  LeftHandPathVector : Inport  Port=5
  RightHandPathVector : Inport  Port=6
  LHVelocity : Inport  Port=7
  RHVelocity : Inport  Port=8
  MidpointPathVector : Inport  Port=9
  MidpointVelocity : Inport  Port=10
  LWAngularVelocityGlobal : Inport  Port=11
  RWAngularVelocityGlobal : Inport  Port=12
  LWristMOFonClub : Inport  Port=13
  RWMOFonClub : Inport  Port=14
  ClubTorqueMagnitude : Sqrt
  Dot Product{,1..4} (5 alike) : DotProduct  OutDataTypeStr=Inherit: Inherit via internal rule
  ForceAlongHandPath : DotProduct  OutDataTypeStr=Inherit: Inherit via internal rule
  HandForceMagnitude : Sqrt
  "LH Work, Impulse, Force on Hand Path" : Subsystem
  LWAngularImpulseonClub : Integrator
  LWAngularWorkonClub : Integrator
  LWFL : nesl_utility/PS-Simulink Converter  PhysicalDomain=network_engine_domain  SubClassName=ps_output  LeftPortType=input  RightPortType=output  PseudoPeriodic=off  Frequencies=[]  VectorFormat=1-D array  Unit=inherit  AffineConversion=off
  LWTG : nesl_utility/PS-Simulink Converter  PhysicalDomain=network_engine_domain  SubClassName=ps_output  LeftPortType=input  RightPortType=output  PseudoPeriodic=off  Frequencies=[]  VectorFormat=1-D array  Unit=inherit  AffineConversion=off
  LinearImpulseonClub : Integrator
  LinearWorkonClub : Integrator
  "RH Work, Impulse, Force on Hand Path" : Subsystem
  RWAngularImpulseonClub : Integrator
  RWAngularWorkonClub : Integrator
  RWFL : nesl_utility/PS-Simulink Converter  PhysicalDomain=network_engine_domain  SubClassName=ps_output  LeftPortType=input  RightPortType=output  PseudoPeriodic=off  Frequencies=[]  VectorFormat=1-D array  Unit=inherit  AffineConversion=off
  RWTG : nesl_utility/PS-Simulink Converter  PhysicalDomain=network_engine_domain  SubClassName=ps_output  LeftPortType=input  RightPortType=output  PseudoPeriodic=off  Frequencies=[]  VectorFormat=1-D array  Unit=inherit  AffineConversion=off
  SumofMomentsLWristonClub : Sum
  SumofMomentsRWristonClub : Sum
  Total Hand Force on Club Global : Sum
  Total Hand Force on Club Local : Sum
  Total Wrist Torque Global : Sum
  Total Wrist Torque Local : Sum
  LWFLocal : PMIOPort  Side=Left
  LWTLocal : PMIOPort  Port=2  Side=Left
  RWTLocal : PMIOPort  Port=3  Side=Left
  RWFLocal : PMIOPort  Port=4  Side=Left
  TotalHandForceGlobal : Outport
  wires:
  RWFL/1 -> Total Hand Force on Club Local/2
  Total Wrist Torque Local/1 -> Dot Product1/1, Dot Product1/2  "TotalWristTorqueLocal"
  LWFL/1 -> Total Hand Force on Club Local/1
  Dot Product/1 -> HandForceMagnitude/1
  Dot Product1/1 -> ClubTorqueMagnitude/1
  Total Hand Force on Club Local/1 -> Dot Product/2, Dot Product/1  "TotalHandForceonClubLocal"
  Total Hand Force on Club Global/1 -> ForceAlongHandPath/1, LinearImpulseonClub/1, Dot Product2/1, TotalHandForceGlobal/1  "TotalHandForceGlobal"
  LWTG/1 -> Total Wrist Torque Local/1
  RWTG/1 -> Total Wrist Torque Local/2
  LWTorqueGlobal/1 -> SumofMomentsLWristonClub/1, Dot Product3/1, Total Wrist Torque Global/1
  LWForceGlobal/1 -> "LH Work, Impulse, Force on Hand Path"/2(LeftHandForceGlobal), Total Hand Force on Club Global/1
  RWForceGlobal/1 -> "RH Work, Impulse, Force on Hand Path"/2(RHForceGlobal), Total Hand Force on Club Global/2
  LeftHandPathVector/1 -> "LH Work, Impulse, Force on Hand Path"/1(LeftHandPathVector)
  RightHandPathVector/1 -> "RH Work, Impulse, Force on Hand Path"/1(RightHandPathVector)
  LHVelocity/1 -> "LH Work, Impulse, Force on Hand Path"/3(LeftHandVelocity)
  RHVelocity/1 -> "RH Work, Impulse, Force on Hand Path"/3(RightHandVelocity)
  MidpointPathVector/1 -> ForceAlongHandPath/2
  Dot Product2/1 -> LinearWorkonClub/1
  MidpointVelocity/1 -> Dot Product2/2
  Dot Product3/1 -> LWAngularWorkonClub/1  "LWonClubAngularPower"
  LWAngularVelocityGlobal/1 -> Dot Product3/2
  Dot Product4/1 -> RWAngularWorkonClub/1  "RWonClubAngularPower"
  RWAngularVelocityGlobal/1 -> Dot Product4/2
  RWTorqueGlobal/1 -> SumofMomentsRWristonClub/1, Dot Product4/1, Total Wrist Torque Global/2
  SumofMomentsLWristonClub/1 -> LWAngularImpulseonClub/1  "SumofMomentsLWristonClub"
  SumofMomentsRWristonClub/1 -> RWAngularImpulseonClub/1  "SumofMomentsRWristonClub"
  LWristMOFonClub/1 -> SumofMomentsLWristonClub/2
  RWMOFonClub/1 -> SumofMomentsRWristonClub/2
  connections:
  LWFLocal/RConn1 -- LWFL/LConn1
  RWFLocal/RConn1 -- RWFL/LConn1
  LWTG/LConn1 -- LWTLocal/RConn1
  RWTLocal/RConn1 -- RWTG/LConn1
